simulink model "astolfi_kin"  (R2021b)
settings: Solver=VariableStepAuto  StartTime=0.0  StopTime=25  RelTol=1e-10
settings Model: Creator=mbober  LastModifiedBy=mbober

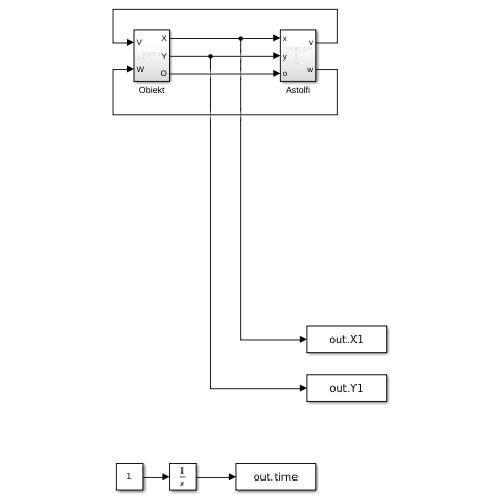
[thumbnail: Simulink's stored preview of the top-level diagram]
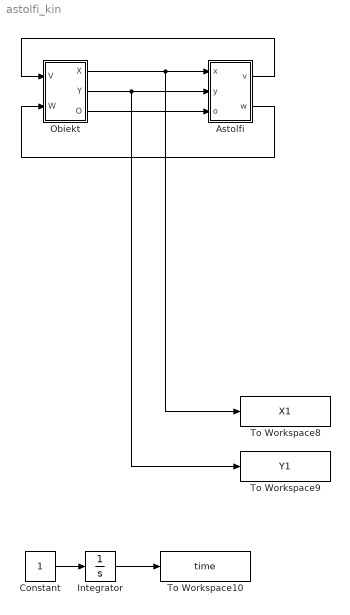
== system astolfi_kin ==
  Astolfi : Subsystem
  Constant : Constant
  Integrator : Integrator
  Obiekt : Subsystem
  To Workspace10 : ToWorkspace  VariableName=time  SampleTime=-1
  To Workspace8 : ToWorkspace  VariableName=X1  SampleTime=-1
  To Workspace9 : ToWorkspace  VariableName=Y1  SampleTime=-1
  wires:
  Obiekt/1(X) -> Astolfi/1(x), To Workspace8/1
  Obiekt/2(Y) -> Astolfi/2(y), To Workspace9/1
  Constant/1 -> Integrator/1
  Integrator/1 -> To Workspace10/1
  Obiekt/3(O) -> Astolfi/3(o)
  Astolfi/1(v) -> Obiekt/1(V)
  Astolfi/2(w) -> Obiekt/2(W)

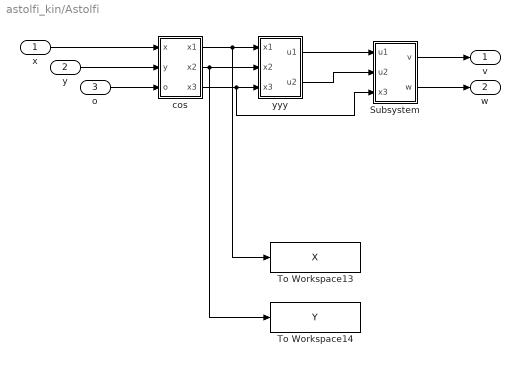
== system astolfi_kin/Astolfi ==
  x : Inport
  y : Inport  Port=2
  o : Inport  Port=3
  Subsystem : Subsystem
  To Workspace13 : ToWorkspace  VariableName=X  SampleTime=-1
  To Workspace14 : ToWorkspace  VariableName=Y  SampleTime=-1
  cos : Subsystem
  yyy : Subsystem
  v : Outport
  w : Outport  Port=2
  wires:
  Subsystem/1(v) -> v/1
  x/1 -> cos/1(x)
  Subsystem/2(w) -> w/1
  y/1 -> cos/2(y)
  o/1 -> cos/3(o)
  cos/3(x3) -> Subsystem/3(x3), yyy/3(x3)
  yyy/2(u2) -> Subsystem/2(u2)
  yyy/1(u1) -> Subsystem/1(u1)
  cos/2(x2) -> yyy/2(x2), To Workspace14/1
  cos/1(x1) -> yyy/1(x1), To Workspace13/1

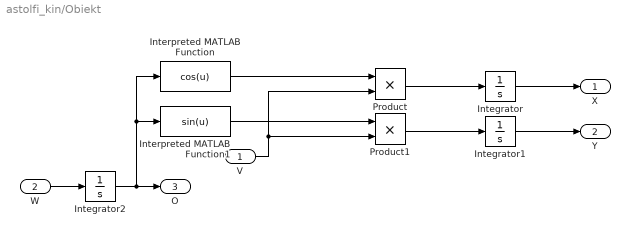
== system astolfi_kin/Obiekt ==
  V : Inport
  W : Inport  Port=2
  Integrator : Integrator  InitialCondition=5
  Integrator1 : Integrator  InitialCondition=6
  Integrator2 : Integrator  InitialCondition=3
  Interpreted MATLAB Function : MATLABFcn  MATLABFcn=cos(u)
  Interpreted MATLAB Function1 : MATLABFcn  MATLABFcn=sin(u)
  Product : Product
  Product1 : Product
  X : Outport
  Y : Outport  Port=2
  O : Outport  Port=3
  wires:
  Product1/1 -> Integrator1/1
  Product/1 -> Integrator/1
  Integrator/1 -> X/1
  Integrator2/1 -> O/1, Interpreted MATLAB Function/1, Interpreted MATLAB Function1/1
  V/1 -> Product1/2, Product/2
  Integrator1/1 -> Y/1
  Interpreted MATLAB Function1/1 -> Product1/1
  W/1 -> Integrator2/1
  Interpreted MATLAB Function/1 -> Product/1

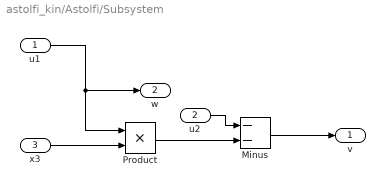
== system astolfi_kin/Astolfi/Subsystem ==
  u1 : Inport
  u2 : Inport  Port=2
  x3 : Inport  Port=3
  Minus : Sum  Inputs=--
  Product : Product
  v : Outport
  w : Outport  Port=2
  wires:
  u2/1 -> Minus/1
  Product/1 -> Minus/2
  x3/1 -> Product/2
  u1/1 -> w/1, Product/1
  Minus/1 -> v/1

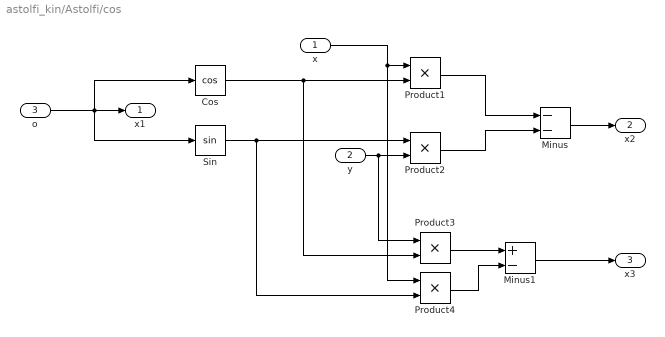
== system astolfi_kin/Astolfi/cos ==
  x : Inport
  y : Inport  Port=2
  o : Inport  Port=3
  Cos : Trigonometry  Operator=cos
  Minus : Sum  Inputs=--
  Minus1 : Sum  Inputs=+-
  Product{1..4} (4 alike) : Product
  Sin : Trigonometry
  x1 : Outport
  x2 : Outport  Port=2
  x3 : Outport  Port=3
  wires:
  o/1 -> Sin/1, Cos/1, x1/1
  Minus/1 -> x2/1
  x/1 -> Product4/1, Product1/1
  Product1/1 -> Minus/1
  y/1 -> Product3/1, Product2/2
  Sin/1 -> Product4/2, Product2/1
  Product2/1 -> Minus/2
  Minus1/1 -> x3/1
  Product3/1 -> Minus1/1
  Product4/1 -> Minus1/2
  Cos/1 -> Product3/2, Product1/2

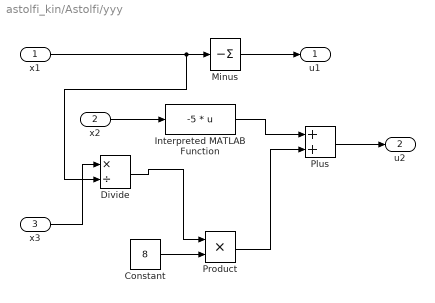
== system astolfi_kin/Astolfi/yyy ==
  x1 : Inport
  x2 : Inport  Port=2
  x3 : Inport  Port=3
  Constant : Constant  Value=8
  Divide : Product  Inputs=*/
  Interpreted MATLAB Function : MATLABFcn  MATLABFcn=-5 * u
  Minus : Sum  Inputs=-
  Plus : Sum
  Product : Product
  u1 : Outport
  u2 : Outport  Port=2
  wires:
  x1/1 -> Divide/2, Minus/1
  Divide/1 -> Product/1
  Minus/1 -> u1/1
  x3/1 -> Divide/1
  x2/1 -> Interpreted MATLAB Function/1
  Plus/1 -> u2/1
  Interpreted MATLAB Function/1 -> Plus/1
  Constant/1 -> Product/2
  Product/1 -> Plus/2
